simulink model "Inner1"  (Simulink 8.7)
settings: Solver=ode45  StartTime=0.0  StopTime=10.0  RelTol=1e-3
settings Model: Creator=scaife  LastModifiedBy=hamza  ExtModeAutoUpdateStatusClock=off
settings DataIOCC: SaveFormat=Structure  SignalLoggingSaveFormat=ModelDataLogs  SignalLoggingName=sigsOut
settings DebuggingCC: SaveWithParameterizedLinksMsg=none  SignalResolutionControl=TryResolveAllWithWarning  MultiTaskDSMMsg=warning  MultiTaskCondExecSysMsg=none
settings HardwareCC: TargetUnknown=on
settings SFSimCC: SimParseCustomCode=off
settings GRTTargetCC: GeneratePreprocessorConditionals=Use local settings  CombineOutputUpdateFcns=off  GRTInterface=on

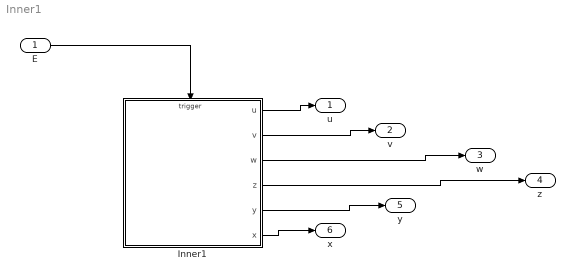
== system Inner1 ==
  E : Inport
  Inner1 : Stateflow chart  TreatAsAtomicUnit=on
  u : Outport
  v : Outport  Port=2
  w : Outport  Port=3
  z : Outport  Port=4
  y : Outport  Port=5
  x : Outport  Port=6
  wires:
  E/1 -> Inner1/Trigger
  Inner1/1(u) -> u/1
  Inner1/2(v) -> v/1
  Inner1/3(w) -> w/1
  Inner1/4(z) -> z/1
  Inner1/5(y) -> y/1
  Inner1/6(x) -> x/1

== stateflow chart Inner1 ==
  state A/
    du: u++;
    state A1/
      en: x+=1;
      du: x+=10;
    state A2/
      en: x+=1000;
      du: x+=10000;
    state A3/
      ex: v+=1000;
      state A3a/
        ex: v+=10000;
      (default) -> A3a
    (default) -> A3
    A -> (junction 8) [order 3] : E[u%%3==2]{w++;}/v++;
    A -> A1 [order 2] : E[u%%3==0]{y++;}/z++;
    A -> A2 [order 1] : E[u%%3==1]
        | {y+=1000;}/z+=1000;
  (default) -> A
  data: u output int32; v output int32; w output int32; z output int32; y output int32; x output int32
  events: E input EITHER_EDGE_EVENT
